simulink model "lotka_volterra_sim"  (R2023b)
settings: Solver=ode45  StartTime=0.0  StopTime=tf  RelTol=1e-5
undefined symbols (not defined in the file): a, b, c, d, x0
settings Model: Creator=miqui  LastModifiedBy=miqui

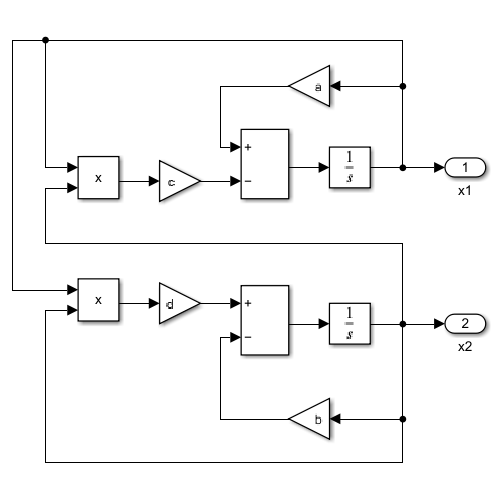
[thumbnail: Simulink's stored preview of the top-level diagram]
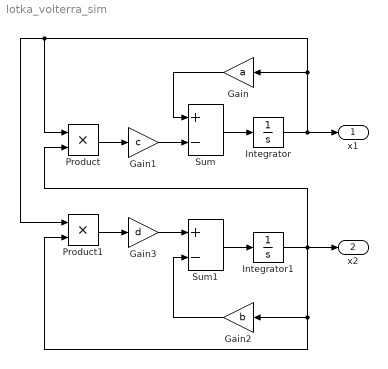
== system lotka_volterra_sim ==
  Gain : Gain  Gain=a
  Gain1 : Gain  Gain=c
  Gain2 : Gain  Gain=b
  Gain3 : Gain  Gain=d
  Integrator : Integrator  InitialCondition=x0(1)
  Integrator1 : Integrator  InitialCondition=x0(2)
  Product : Product
  Product1 : Product
  Sum : Sum  Inputs=+-
  Sum1 : Sum  Inputs=+-
  x1 : Outport
  x2 : Outport  Port=2
  wires:
  Sum/1 -> Integrator/1
  Integrator/1 -> x1/1, Gain/1, Product/1, Product1/1
  Gain/1 -> Sum/1
  Product/1 -> Gain1/1
  Gain1/1 -> Sum/2
  Sum1/1 -> Integrator1/1
  Integrator1/1 -> x2/1, Product/2, Gain2/1, Product1/2
  Gain2/1 -> Sum1/2
  Gain3/1 -> Sum1/1
  Product1/1 -> Gain3/1
